simulink model "Pid_ZOH"  (R2021a)
settings: Solver=ode45  StartTime=0.0  StopTime=2  RelTol=1e-3
undefined symbols (not defined in the file): daq, drv, est_par, gbox, mot, rads2rpm, sens, T_samp, zoh_den, zoh_num
settings Model: Creator=gioel  LastModifiedBy=gioel
settings DataIOCC: ReturnWorkspaceOutputs=off

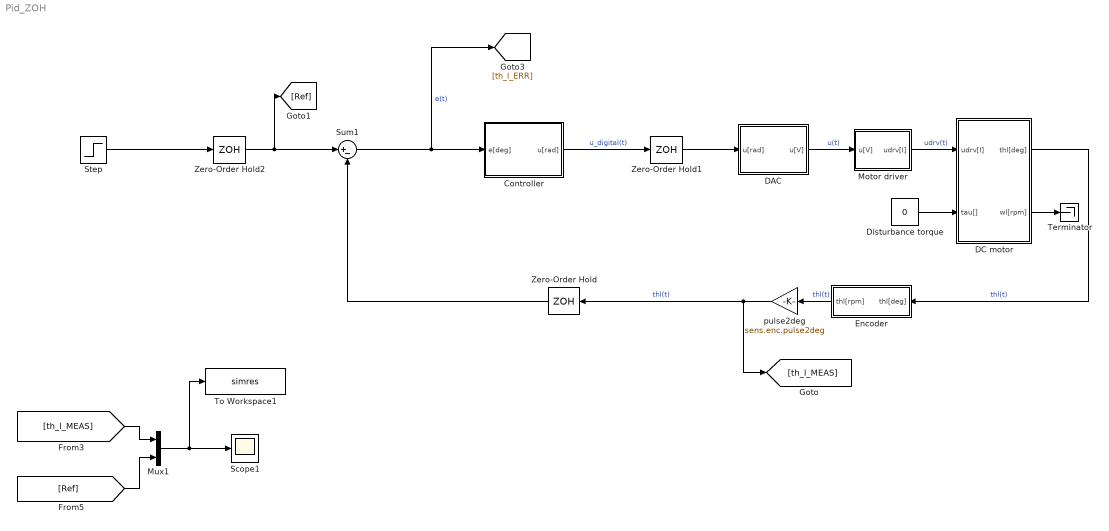
== system Pid_ZOH ==
  Controller : Subsystem
  DAC : Subsystem
  DC motor : Subsystem
  Disturbance torque : Constant  Value=0
  Encoder : Subsystem
  Motor driver : Subsystem
  Mux1 : Mux  Inputs=2
  Scope1 : Scope
  Step : Step  Time=0  After=50  SampleTime=0
  Sum1 : Sum  Inputs=|+-
  Terminator : Terminator
  To Workspace1 : ToWorkspace  VariableName=simres  SaveFormat=Structure With Time  SampleTime=-1
  Zero-Order Hold : ZeroOrderHold  SampleTime=T_samp
  Zero-Order Hold1 : ZeroOrderHold  SampleTime=T_samp
  Zero-Order Hold2 : ZeroOrderHold  SampleTime=T_samp
  pulse2deg : Gain  Gain=sens.enc.pulse2deg
  wires:
  DAC/1(u[V]) -> Motor driver/1(u[V])  "u(t)"
  Zero-Order Hold2/1 -> [Ref], Sum1/1
  Sum1/1 -> [th_l_ERR], Controller/1(e[deg])  "e(t)"
  Motor driver/1(udrv[I]) -> DC motor/1(udrv[I])  "udrv(t)"
  DC motor/1(thl[deg]) -> Encoder/1(thl[deg])  "thl(t)"
  pulse2deg/1 -> Zero-Order Hold/1, [th_l_MEAS]  "thl(t)"
  [th_l_MEAS] -> Mux1/1
  Encoder/1(thl[rpm]) -> pulse2deg/1  "thl(t)"
  Disturbance torque/1 -> DC motor/2(tau[])
  DC motor/2(wl[rpm]) -> Terminator/1
  Controller/1(u[rad]) -> Zero-Order Hold1/1  "u_digital(t)"
  Zero-Order Hold1/1 -> DAC/1(u[rad])
  Step/1 -> Zero-Order Hold2/1
  Mux1/1 -> Scope1/1, To Workspace1/1
  [Ref] -> Mux1/2
  Zero-Order Hold/1 -> Sum1/2

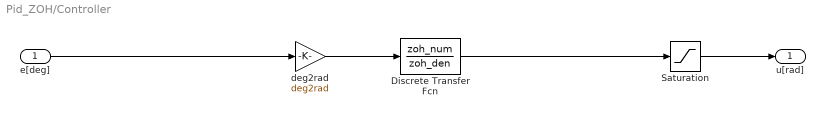
== system Pid_ZOH/Controller ==
  e[deg] : Inport  Unit=deg
  Discrete Transfer Fcn : DiscreteTransferFcn  Numerator=zoh_num  Denominator=zoh_den
  Saturation : Saturate  UpperLimit=daq.dac.vdd  LowerLimit=daq.dac.vss
  deg2rad : Gain  Gain=deg2rad
  u[rad] : Outport
  wires:
  e[deg]/1 -> deg2rad/1
  Saturation/1 -> u[rad]/1
  Discrete Transfer Fcn/1 -> Saturation/1
  deg2rad/1 -> Discrete Transfer Fcn/1

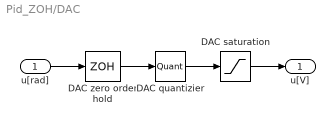
== system Pid_ZOH/DAC ==
  u[rad] : Inport
  DAC quantizier : Quantizer  QuantizationInterval=daq.dac.q
  DAC saturation : Saturate  UpperLimit=10  LowerLimit=-10
  DAC zero order hold : ZeroOrderHold  SampleTime=sens.enc.T_s
  u[V] : Outport
  wires:
  DAC quantizier/1 -> DAC saturation/1
  DAC zero order hold/1 -> DAC quantizier/1
  DAC saturation/1 -> u[V]/1
  u[rad]/1 -> DAC zero order hold/1

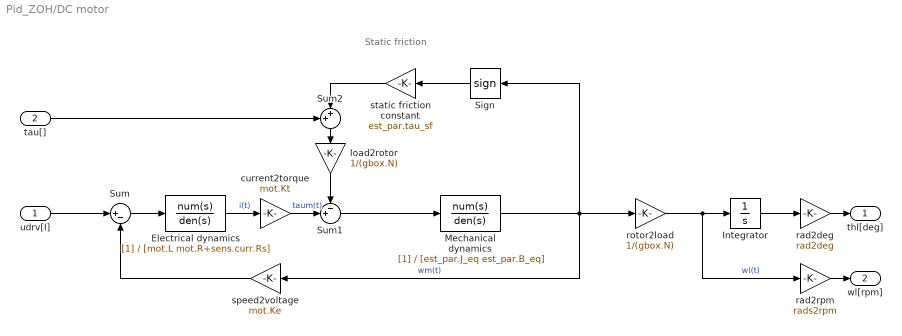
== system Pid_ZOH/DC motor ==
  note: Static friction
  udrv[I] : Inport  Unit=V
  tau[] : Inport  Port=2  Unit=V
  Electrical dynamics : TransferFcn  Denominator=[mot.L mot.R+sens.curr.Rs]
  Integrator : Integrator
  Mechanical dynamics : TransferFcn  Denominator=[est_par.J_eq est_par.B_eq]
  Sign : Signum  ZeroCross=off
  Sum : Sum  Inputs=|+-
  Sum1 : Sum  Inputs=-+|
  Sum2 : Sum  Inputs=++|
  current2torque : Gain  Gain=mot.Kt
  load2rotor : Gain  Gain=1/(gbox.N)
  rad2deg : Gain  Gain=rad2deg
  rad2rpm : Gain  Gain=rads2rpm
  rotor2load : Gain  Gain=1/(gbox.N)
  speed2voltage : Gain  Gain=mot.Ke
  static friction constant : Gain  Gain=est_par.tau_sf
  thl[deg] : Outport  Unit=deg
  wl[rpm] : Outport  Port=2  Unit=rpm
  wires:
  load2rotor/1 -> Sum1/1
  Mechanical dynamics/1 -> Sign/1, rotor2load/1, speed2voltage/1  "wm(t)"
  Sign/1 -> static friction constant/1
  current2torque/1 -> Sum1/2  "taum(t)"
  Sum1/1 -> Mechanical dynamics/1
  speed2voltage/1 -> Sum/2
  rotor2load/1 -> rad2rpm/1, Integrator/1  "wl(t)"
  Electrical dynamics/1 -> current2torque/1  "i(t)"
  Integrator/1 -> rad2deg/1
  Sum/1 -> Electrical dynamics/1
  rad2rpm/1 -> wl[rpm]/1
  rad2deg/1 -> thl[deg]/1
  udrv[I]/1 -> Sum/1
  static friction constant/1 -> Sum2/2
  Sum2/1 -> load2rotor/1
  tau[]/1 -> Sum2/1

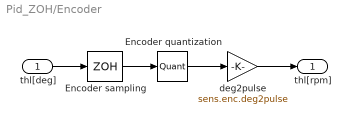
== system Pid_ZOH/Encoder ==
  thl[deg] : Inport
  Encoder quantization : Quantizer  QuantizationInterval=sens.enc.q
  Encoder sampling : ZeroOrderHold  SampleTime=sens.enc.T_s
  deg2pulse : Gain  Gain=sens.enc.deg2pulse
  thl[rpm] : Outport
  wires:
  Encoder quantization/1 -> deg2pulse/1
  deg2pulse/1 -> thl[rpm]/1
  Encoder sampling/1 -> Encoder quantization/1
  thl[deg]/1 -> Encoder sampling/1

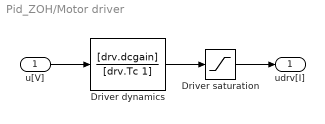
== system Pid_ZOH/Motor driver ==
  u[V] : Inport
  Driver dynamics : TransferFcn  Numerator=[drv.dcgain]  Denominator=[drv.Tc 1]
  Driver saturation : Saturate  UpperLimit=12  LowerLimit=-12
  udrv[I] : Outport
  wires:
  Driver saturation/1 -> udrv[I]/1
  Driver dynamics/1 -> Driver saturation/1
  u[V]/1 -> Driver dynamics/1
